simulink model "PD_continouse_Servo_sine_input_final"  (R2022a)
settings: Solver=ode4  StartTime=0.0  StopTime=10.0  FixedStep=0.001  RelTol=1e-3
libraries: slpidlib x1
settings Model: Creator=acer  LastModifiedBy=Electronica Care
settings SolverCC: AlgebraicLoopSolver=TrustRegion
settings DebuggingCC: SFMachineParentedDataDiag=warning  ArithmeticOperatorsInVariantConditions=warning
settings ModelReferenceCC: EnableRefExpFcnMdlSchedulingChecks=off
settings SFSimCC: CustomCodeUndefinedFunction=UseInterfaceOnly
settings RTWCC: Description=Generic Real-Time Target

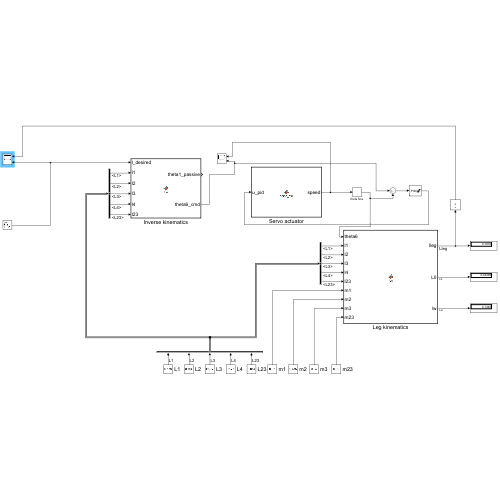
[thumbnail: Simulink's stored preview of the top-level diagram]
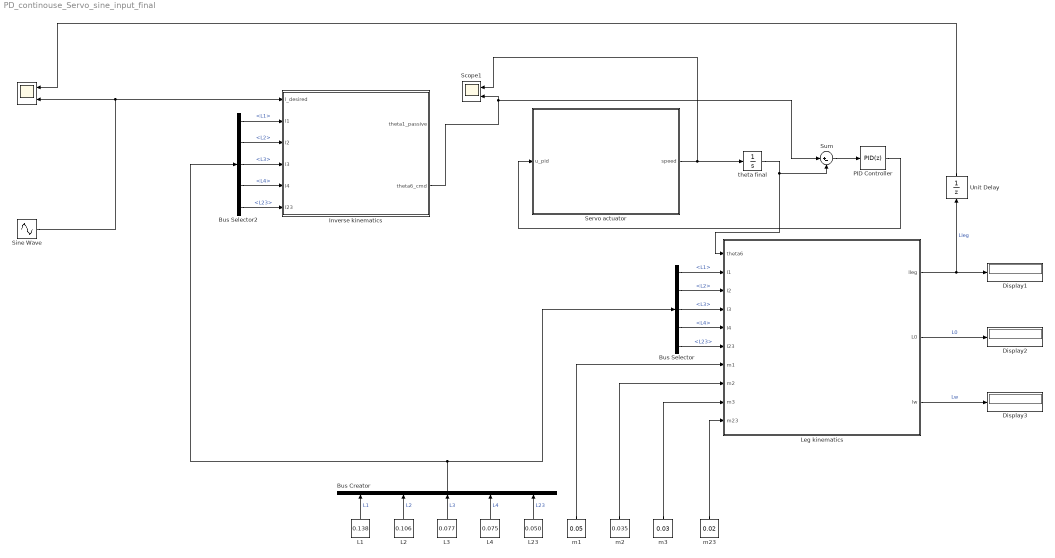
== system PD_continouse_Servo_sine_input_final ==
  " " : Scope  NumInputPorts=2
  Bus Creator : BusCreator  Inputs=5
  Bus Selector : BusSelector  OutputSignals=L1,L2,L3,L4,L23
  Bus Selector2 : BusSelector  OutputSignals=L1,L2,L3,L4,L23
  Display1 : Display
  Display2 : Display
  Display3 : Display
  Inverse kinematics : MATLAB Function  TreatAsAtomicUnit=on
  L1 : Constant  Value=0.138
  L2 : Constant  Value=0.106
  L23 : Constant  Value=0.050
  L3 : Constant  Value=0.077
  L4 : Constant  Value=0.075
  Leg kinematics : MATLAB Function  TreatAsAtomicUnit=on
  PID Controller : slpidlib/PID Controller  Controller=PID  Form=Parallel  TimeDomain=Discrete-time  UseExternalTs=off  SampleTime=0.001  IntegratorMethod=Forward Euler  FilterMethod=Forward Euler  ControllerParametersSource=internal  P=50  I=2000  UseKiTs=off  D=1  N=1000  UseFilter=on  TunerSelectOption=Transfer Function Based (PID Tuner App)  InitialConditionSource=internal  InitialConditionForIntegrator=100  InitialConditionForFilter=0  DifferentiatorICPrevScaledInput=0  ExternalReset=none  TrackingMode=off  Kt=1  LimitOutput=on  SatLimitsSource=internal  UpperSaturationLimit=100  LowerSaturationLimit=-100  LinearizeAsGain=on  AntiWindupMode=clamping  Kb=1  POutMin=[]  POutMax=[]  IOutMin=[]  IOutMax=[]  DOutMin=[]  DOutMax=[]  NOutMin=[]  NOutMax=[]  SumOutMin=[]  SumOutMax=[]  SaturationOutMin=[]  SaturationOutMax=[]  PParamMin=[]  PParamMax=[]  IParamMin=[]  IParamMax=[]  DParamMin=[]  DParamMax=[]  NParamMin=[]  NParamMax=[]  KbParamMin=[]  KbParamMax=[]  KtParamMin=[]  KtParamMax=[]  KbOutMin=[]  KbOutMax=[]  KtOutMin=[]  KtOutMax=[]  IntegratorOutMin=[]  IntegratorOutMax=[]  FilterOutMin=[]  FilterOutMax=[]  SumI1OutMin=[]  SumI1OutMax=[]  SumI2OutMin=[]  SumI2OutMax=[]  SumI3OutMin=[]  SumI3OutMax=[]  SumI4OutMin=[]  SumI4OutMax=[]  SumDOutMin=[]  SumDOutMax=[]  DifferentiatorOutMin=[]  DifferentiatorOutMax=[]  FilterDiffOutCoefMin=[]  FilterDiffOutCoefMax=[]  ReciprocalOutMin=[]  ReciprocalOutMax=[]  SumDenOutMin=[]  SumDenOutMax=[]  SumNumOutMin=[]  SumNumOutMax=[]  DivideOutMin=[]  DivideOutMax=[]  UdiffTsProdOutMin=[]  UdiffTsProdOutMax=[]  NTsProdOutMin=[]  NTsProdOutMax=[]  UintegralTsProdOutMin=[]  UintegralTsProdOutMax=[]  UngainTsProdOutMin=[]  UngainTsProdOutMax=[]  IntegratorContinuousStateAttributes=''  IntegratorStateMustResolveToSignalObject=off  IntegratorRTWStateStorageClass=Auto  FilterContinuousStateAttributes=''  FilterStateMustResolveToSignalObject=off  FilterRTWStateStorageClass=Auto  ParallelPVariant=InternalParameters  IdealPVariant=Disabled  IVariant=InternalParameters  DVariant=InternalParameters  IntegratorVariant=Discrete  SatVariant=Enabled  AWVariant=DiscClampingParallel  PCopyVariant=Disabled  TRVariant=Disabled  FdbkBlocksVariant=Forward  IdealPFdbkVariant=Disabled  SatFdbkVariant=Disabled  DerivativeFilterVariant=ForwardEulerFilter  NVariant=InternalParameters  NCopyVariant=Disabled  FilterICVariant=InternalICsFilter  IntegratorICVariant=InternalICs  ExternalResetVariant=Disabled  TRSumVariant=Passthrough  SumFdbkVariant=Disabled  SumVariant=Sum_PID  TsampFilterVariant=InternalTs  TsampNgainVariant=Passthrough  TsampIntegralVariant=Passthrough  ExternalSaturationOutDataTypeStr=Inherit: Same as second input  aMode=0
  Scope1 : Scope  NumInputPorts=2
  Servo actuator : MATLAB Function  TreatAsAtomicUnit=on  SystemSampleTime=0.001
  Sine Wave : Sin  Amplitude=0.03  Bias=0.15  SampleTime=0
  Sum : Sum  Inputs=|+-
  Unit Delay : UnitDelay  InitialCondition=0.11  SampleTime=0.001  HasFrameUpgradeWarning=on
  m1 : Constant  Value=0.05
  m2 : Constant  Value=0.035
  m23 : Constant  Value=0.02
  m3 : Constant  Value=0.03
  theta final : Integrator
  wires:
  Servo actuator/1(speed) -> theta final/1, Scope1/1
  Leg kinematics/1(lleg) -> Display1/1, Unit Delay/1  "Lleg"
  m1/1 -> Leg kinematics/7(m1)
  m2/1 -> Leg kinematics/8(m2)
  m3/1 -> Leg kinematics/9(m3)
  m23/1 -> Leg kinematics/10(m23)
  Leg kinematics/2(L0) -> Display2/1  "L0"
  Leg kinematics/3(lw) -> Display3/1  "Lw"
  Bus Selector/3 -> Leg kinematics/4(l3)  "<L3>"
  Bus Selector/2 -> Leg kinematics/3(l2)  "<L2>"
  Bus Selector/1 -> Leg kinematics/2(l1)  "<L1>"
  Bus Selector/4 -> Leg kinematics/5(l4)  "<L4>"
  Bus Selector/5 -> Leg kinematics/6(l23)  "<L23>"
  L3/1 -> Bus Creator/3  "L3"
  L2/1 -> Bus Creator/2  "L2"
  L1/1 -> Bus Creator/1  "L1"
  L4/1 -> Bus Creator/4  "L4"
  L23/1 -> Bus Creator/5  "L23"
  Bus Selector2/1 -> Inverse kinematics/2(l1)  "<L1>"
  Bus Selector2/2 -> Inverse kinematics/3(l2)  "<L2>"
  Bus Selector2/3 -> Inverse kinematics/4(l3)  "<L3>"
  Bus Selector2/4 -> Inverse kinematics/5(l4)  "<L4>"
  Bus Selector2/5 -> Inverse kinematics/6(l23)  "<L23>"
  Bus Creator/1 -> Bus Selector/1, Bus Selector2/1
  Sine Wave/1 -> Inverse kinematics/1(l_desired), " "/2
  Inverse kinematics/2(theta6_cmd) -> Sum/1, Scope1/2
  Unit Delay/1 -> " "/1
  theta final/1 -> Sum/2, Leg kinematics/1(theta6)
  Sum/1 -> PID Controller/1
  PID Controller/1 -> Servo actuator/1(u_pid)

== matlab function PD_continouse_Servo_sine_input_final/Inverse kinematics ==
  data: l_desired input; theta1_passive output; l1 input; l2 input; l3 input; l4 input; l23 input; theta6_cmd output
function [theta1_passive, theta6_cmd] = fcn(l_desired, l1, l2, l3, l4, l23)
    % 1. تأمين الدخل
    l_desired = max(min(l_desired, (l1+l2)-0.01), 0.05); 

    % 2. حساب theta1_passive (الزاوية الحرة في الهيب)
    % في التصميم ده، theta1 هي اللي بتحدد الارتفاع الأساسي
    arg1 = (l_desired^2 + l2^2 - l1^2) / (2 * l_desired * l2);
    theta1_passive = asin(max(min(arg1, 1), -1));
    
    % 3. حساب l5 (الوتر اللي بيقفل الميكانيزم الرباعي)
    l5_sq = l2^2 + l4^2 - 2*l2*l4*cos(theta1_passive + pi/4);
    l5 = sqrt(max(l5_sq, 0.0001));
    
    % 4. حساب theta6_cmd (زاوية السيرفو عند الركبة)
    % دي الزاوية اللي لازم السيرفو يروحلها عشان يحافظ على اتزان الشكل الرباعي
    cos_theta6 = (l3^2 + l23^2 - l5^2) / (2 * l3 * l23);
    theta6_cmd = acos(max(min(cos_theta6, 1), -1));
end

== matlab function PD_continouse_Servo_sine_input_final/Servo actuator ==
  data: u_pid input; speed output
function speed = servo_ctrl(u_pid)
    % u_pid هو مخرج بلوك الـ PID الخارجي
    speed = u_pid;
    
    % نفس الـ Limiter اللي كان في كودك الأصلي
    if speed > 15
        speed = 15;
    elseif speed < -15
        speed = -15;
    end
end

== matlab function PD_continouse_Servo_sine_input_final/Leg kinematics ==
  data: theta6 input; lleg output; l1 input; l2 input; l3 input; l4 input; l23 input; m1 input; m2 input; m3 input; m23 input; L0 output; lw output
function [lleg, L0, lw] = fcn(theta6, l1, l2, l3, l4, l23, m1, m2, m3, m23)
    % 1. حساب الوتر l5 بناءً على وضع السيرفو الحالي
    l5_sq = l3^2 + l23^2 - 2 * l3 * l23 * cos(theta6);
    l5 = sqrt(max(l5_sq, 0.0001)); 

    % 2. حساب theta1 (الزاوية الناتجة عن حركة الميكانيزم)
    arg_t1 = (l2^2 + l4^2 - l5^2) / (2 * l2 * l4);
    theta1 = acos(max(min(arg_t1, 1), -1)) - pi/4;

    % 3. حساب theta4 (زاوية اللينك السفلي) لغلق الشكل
    arg_t2 = (l4 * sin(theta1 + pi/4)) / l5;
    theta2 = asin(max(min(arg_t2, 1), -1));
    
    arg_t3 = (l23^2 + l5^2 - l3^2) / (2 * l23 * l5);
    theta3 = acos(max(min(arg_t3, 1), -1));
    
    theta4 = pi - theta1 - theta2 - theta3;

    % 4. طول الرجل الفعلي (المخرج الأساسي للسكوب)
    lleg = l2 * sin(theta1) + l1 * sin(theta4);

    % حسابات مركز الثقل (تظل كما هي لضمان الاتزان)
    xc2 = (l2 * sin(theta1)) / 2;
    xc1 = l2 * sin(theta1) + (l1 * sin(pi - theta4)) / 2;
    M_total = m1 + m2 + m3 + m23;
    L0 = (m1*xc1 + m2*xc2) / max(M_total, 0.01); % تبسيط للمناقشة
    lw = lleg - L0;
end
